simulink model "aclarke_park_trans"  (R2015a)
settings: Solver=ode45  StartTime=0.0  StopTime=40/1000  RelTol=1e-3
settings Model: Creator=Windows 10  LastModifiedBy=Windows 10

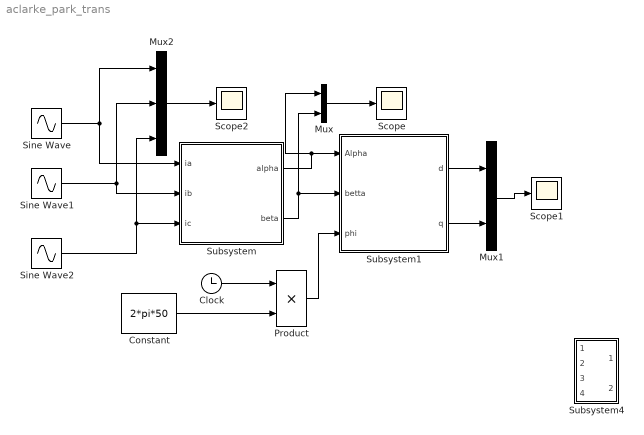
== system aclarke_park_trans ==
  Clock : Clock
  Constant : Constant  Value=2*pi*50
  Mux : Mux  Inputs=2
  Mux1 : Mux  Inputs=2
  Mux2 : Mux  Inputs=3
  Product : Product
  Scope : Scope
  Scope1 : Scope
  Scope2 : Scope
      settings: SaveName=ScopeData2
  Sine Wave : Sin  Amplitude=180  Frequency=50*2*pi  SampleTime=0
  Sine Wave1 : Sin  Amplitude=180  Frequency=50*2*pi  Phase=-2*pi/3  SampleTime=0
  Sine Wave2 : Sin  Amplitude=180  Frequency=50*2*pi  Phase=2*pi/3  SampleTime=0
  Subsystem : Subsystem
  Subsystem1 : Subsystem
  Subsystem4 : Subsystem
  wires:
  Mux1/1 -> Scope1/1
  Mux/1 -> Scope/1
  Subsystem/1(alpha) -> Mux/1, Subsystem1/1(Alpha)
  Subsystem/2(beta) -> Mux/2, Subsystem1/2(betta)
  Subsystem1/1(d) -> Mux1/1
  Subsystem1/2("q ") -> Mux1/2
  Mux2/1 -> Scope2/1
  Sine Wave/1 -> Mux2/1, Subsystem/1(ia)
  Sine Wave2/1 -> Mux2/3, Subsystem/3(ic)
  Sine Wave1/1 -> Subsystem/2(ib), Mux2/2
  Product/1 -> Subsystem1/3("phi ")
  Clock/1 -> Product/1
  Constant/1 -> Product/2

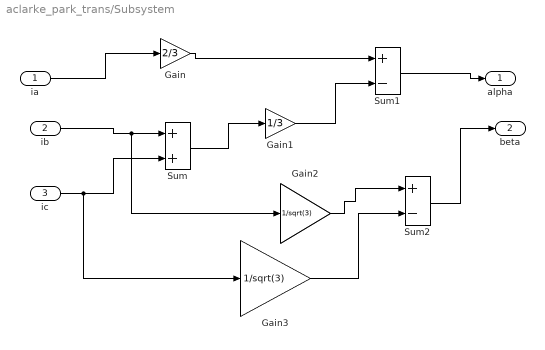
== system aclarke_park_trans/Subsystem ==
  ia : Inport
  ib : Inport  Port=2
  ic : Inport  Port=3
  Gain : Gain  Gain=2/3
  Gain1 : Gain  Gain=1/3
  Gain2 : Gain  Gain=1/sqrt(3)
  Gain3 : Gain  Gain=1/sqrt(3)
  Sum : Sum
  Sum1 : Sum  Inputs=+-
  Sum2 : Sum  Inputs=+-
  alpha : Outport
  beta : Outport  Port=2
  wires:
  Sum1/1 -> alpha/1
  Sum2/1 -> beta/1
  Gain/1 -> Sum1/1
  Gain1/1 -> Sum1/2
  Sum/1 -> Gain1/1
  ia/1 -> Gain/1
  ib/1 -> Gain2/1, Sum/1
  ic/1 -> Gain3/1, Sum/2
  Gain2/1 -> Sum2/1
  Gain3/1 -> Sum2/2

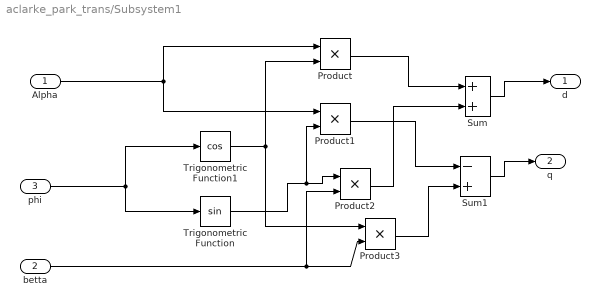
== system aclarke_park_trans/Subsystem1 ==
  Alpha : Inport
  betta : Inport  Port=2
  "phi " : Inport  Port=3
  Product{,1..3} (4 alike) : Product
  Sum : Sum
  Sum1 : Sum  Inputs=-+
  Trigonometric Function : Trigonometry
  Trigonometric Function1 : Trigonometry  Operator=cos
  d : Outport
  "q " : Outport  Port=2
  wires:
  Sum/1 -> d/1
  Sum1/1 -> "q "/1
  "phi "/1 -> Trigonometric Function/1, Trigonometric Function1/1
  Product/1 -> Sum/1
  Product1/1 -> Sum1/1
  Product2/1 -> Sum/2
  Product3/1 -> Sum1/2
  betta/1 -> Product2/2, Product3/2
  Trigonometric Function/1 -> Product1/2, Product2/1
  Trigonometric Function1/1 -> Product3/1, Product/2
  Alpha/1 -> Product1/1, Product/1

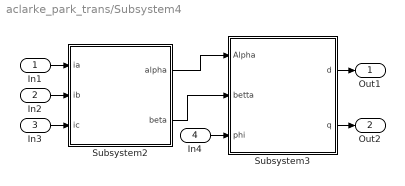
== system aclarke_park_trans/Subsystem4 ==
  In1 : Inport
  In2 : Inport  Port=2
  In3 : Inport  Port=3
  In4 : Inport  Port=4
  Subsystem2 : Subsystem
  Subsystem3 : Subsystem
  Out1 : Outport
  Out2 : Outport  Port=2
  wires:
  Subsystem2/2(beta) -> Subsystem3/2(betta)
  In1/1 -> Subsystem2/1(ia)
  Subsystem3/2("q ") -> Out2/1
  In2/1 -> Subsystem2/2(ib)
  In4/1 -> Subsystem3/3("phi ")
  Subsystem3/1(d) -> Out1/1
  In3/1 -> Subsystem2/3(ic)
  Subsystem2/1(alpha) -> Subsystem3/1(Alpha)

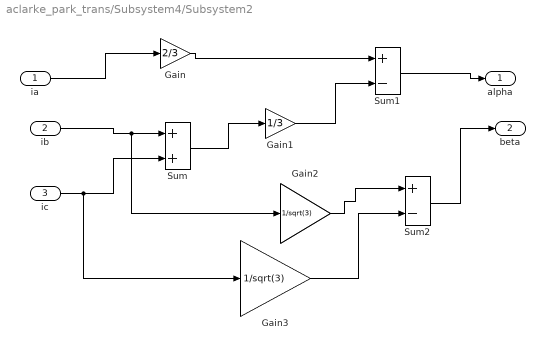
== system aclarke_park_trans/Subsystem4/Subsystem2 ==
  ia : Inport
  ib : Inport  Port=2
  ic : Inport  Port=3
  Gain : Gain  Gain=2/3
  Gain1 : Gain  Gain=1/3
  Gain2 : Gain  Gain=1/sqrt(3)
  Gain3 : Gain  Gain=1/sqrt(3)
  Sum : Sum
  Sum1 : Sum  Inputs=+-
  Sum2 : Sum  Inputs=+-
  alpha : Outport
  beta : Outport  Port=2
  wires:
  Gain3/1 -> Sum2/2
  Gain2/1 -> Sum2/1
  ic/1 -> Sum/2, Gain3/1
  ib/1 -> Sum/1, Gain2/1
  ia/1 -> Gain/1
  Sum/1 -> Gain1/1
  Gain1/1 -> Sum1/2
  Gain/1 -> Sum1/1
  Sum2/1 -> beta/1
  Sum1/1 -> alpha/1

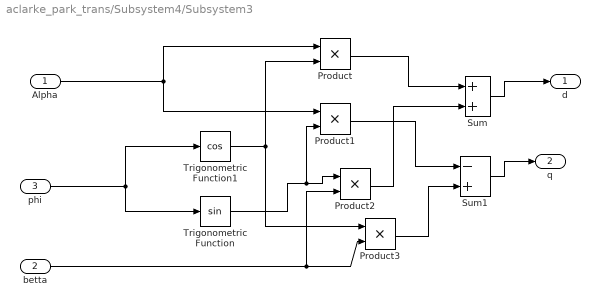
== system aclarke_park_trans/Subsystem4/Subsystem3 ==
  Alpha : Inport
  betta : Inport  Port=2
  "phi " : Inport  Port=3
  Product{,1..3} (4 alike) : Product
  Sum : Sum
  Sum1 : Sum  Inputs=-+
  Trigonometric Function : Trigonometry
  Trigonometric Function1 : Trigonometry  Operator=cos
  d : Outport
  "q " : Outport  Port=2
  wires:
  Alpha/1 -> Product/1, Product1/1
  Trigonometric Function1/1 -> Product/2, Product3/1
  Trigonometric Function/1 -> Product2/1, Product1/2
  betta/1 -> Product3/2, Product2/2
  Product3/1 -> Sum1/2
  Product2/1 -> Sum/2
  Product1/1 -> Sum1/1
  Product/1 -> Sum/1
  "phi "/1 -> Trigonometric Function1/1, Trigonometric Function/1
  Sum1/1 -> "q "/1
  Sum/1 -> d/1
